simulink model "TST_PT_Grip"  (R2016b)
settings: Solver=FixedStepDiscrete  StartTime=0.0  StopTime=simTime  FixedStep=sampleTime  RelTol=1e-3
values from neighbouring files (symbols this model uses):
  testCase = 1    [initTST_PT_Grip_001.m]    (also in initTST_PT_Grip_002.m = 2)
libraries: simulink x9, UnitTest_Lib x6
settings Model: Creator=zhengjinyan  LastModifiedBy=zhengjinyan
settings DebuggingCC: SignalRangeChecking=error

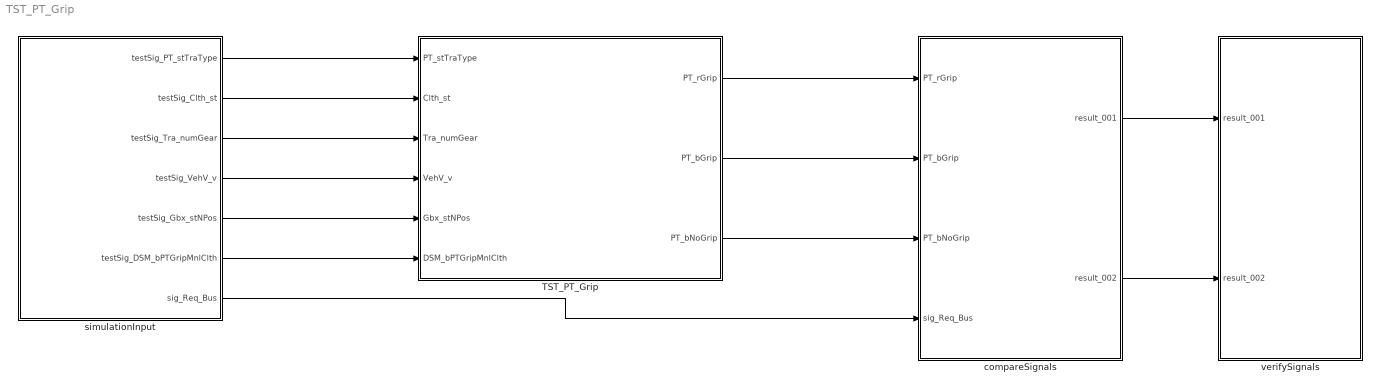
== system TST_PT_Grip ==
  TST_PT_Grip : Subsystem
  compareSignals : Subsystem
  simulationInput : Subsystem
  verifySignals : Subsystem
  wires:
  simulationInput/1(testSig_PT_stTraType) -> TST_PT_Grip/1(PT_stTraType)
  simulationInput/2(testSig_Clth_st) -> TST_PT_Grip/2(Clth_st)
  simulationInput/3(testSig_Tra_numGear) -> TST_PT_Grip/3(Tra_numGear)
  simulationInput/4(testSig_VehV_v) -> TST_PT_Grip/4(VehV_v)
  simulationInput/5(testSig_Gbx_stNPos) -> TST_PT_Grip/5(Gbx_stNPos)
  simulationInput/6(testSig_DSM_bPTGripMnlClth) -> TST_PT_Grip/6(DSM_bPTGripMnlClth)
  TST_PT_Grip/1(PT_rGrip) -> compareSignals/1(PT_rGrip)
  TST_PT_Grip/2(PT_bGrip) -> compareSignals/2(PT_bGrip)
  TST_PT_Grip/3(PT_bNoGrip) -> compareSignals/3(PT_bNoGrip)
  simulationInput/7(sig_Req_Bus) -> compareSignals/4(sig_Req_Bus)
  compareSignals/1(result_001) -> verifySignals/1(result_001)
  compareSignals/2(result_002) -> verifySignals/2(result_002)

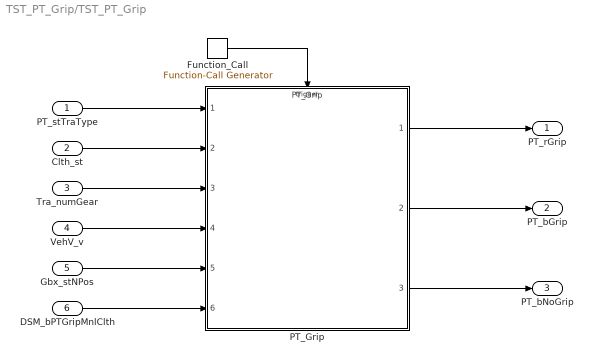
== system TST_PT_Grip/TST_PT_Grip ==
  PT_stTraType : Inport
  Clth_st : Inport  Port=2
  Tra_numGear : Inport  Port=3
  VehV_v : Inport  Port=4
  Gbx_stNPos : Inport  Port=5
  DSM_bPTGripMnlClth : Inport  Port=6
  Function_Call : simulink/Ports & Subsystems/Function-Call Generator  sample_time=sampleTime  numberOfIterations=1
  PT_Grip : ModelReference  ModelNameDialog=PT_Grip  SimulationMode=Normal  ModelReferenceVersion=1.20  TriggerPortName=function  TriggerPortTriggerType=function-call  TriggerPortStatesWhenEnabling=held
  PT_rGrip : Outport
  PT_bGrip : Outport  Port=2
  PT_bNoGrip : Outport  Port=3
  wires:
  Function_Call/1 -> PT_Grip/Trigger
  PT_stTraType/1 -> PT_Grip/1
  Clth_st/1 -> PT_Grip/2
  Tra_numGear/1 -> PT_Grip/3
  VehV_v/1 -> PT_Grip/4
  Gbx_stNPos/1 -> PT_Grip/5
  DSM_bPTGripMnlClth/1 -> PT_Grip/6
  PT_Grip/1 -> PT_rGrip/1
  PT_Grip/2 -> PT_bGrip/1
  PT_Grip/3 -> PT_bNoGrip/1

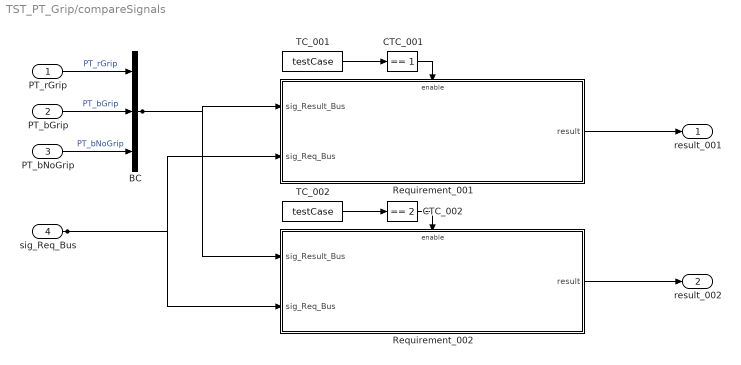
== system TST_PT_Grip/compareSignals ==
  PT_rGrip : Inport
  PT_bGrip : Inport  Port=2
  PT_bNoGrip : Inport  Port=3
  sig_Req_Bus : Inport  Port=4
  BC : BusCreator  Inputs=3
  CTC_001 : simulink/Logic and Bit Operations/Compare To Constant  relop===  const=1  OutDataTypeStr=boolean
  CTC_002 : simulink/Logic and Bit Operations/Compare To Constant  relop===  const=2  OutDataTypeStr=boolean
  Requirement_001 : Subsystem
  Requirement_002 : Subsystem
  TC_001 : Constant  Value=testCase
  TC_002 : Constant  Value=testCase
  result_001 : Outport
  result_002 : Outport  Port=2
  wires:
  PT_rGrip/1 -> BC/1  "PT_rGrip"
  PT_bGrip/1 -> BC/2  "PT_bGrip"
  PT_bNoGrip/1 -> BC/3  "PT_bNoGrip"
  TC_001/1 -> CTC_001/1
  CTC_001/1 -> Requirement_001/Enable
  sig_Req_Bus/1 -> Requirement_001/2(sig_Req_Bus), Requirement_002/2(sig_Req_Bus)
  BC/1 -> Requirement_001/1(sig_Result_Bus), Requirement_002/1(sig_Result_Bus)
  Requirement_001/1(result) -> result_001/1
  TC_002/1 -> CTC_002/1
  CTC_002/1 -> Requirement_002/Enable
  Requirement_002/1(result) -> result_002/1

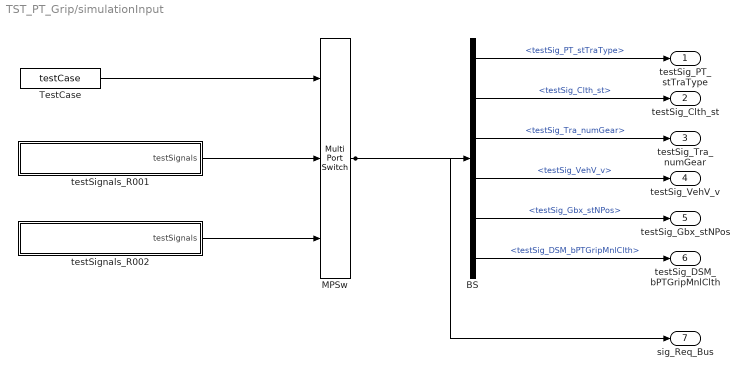
== system TST_PT_Grip/simulationInput ==
  BS : BusSelector  OutputSignals=testSig_PT_stTraType,testSig_Clth_st,testSig_Tra_numGear,testSig_VehV_v,testSig_Gbx_stNPos,testSig_DSM_bPTGripMnlClth
  MPSw : MultiPortSwitch  Inputs=2  SaturateOnIntegerOverflow=on  InputSameDT=on
  TestCase : Constant  Value=testCase
  testSignals_R001 : Subsystem
  testSignals_R002 : Subsystem
  testSig_PT_stTraType : Outport
  testSig_Clth_st : Outport  Port=2
  testSig_Tra_numGear : Outport  Port=3
  testSig_VehV_v : Outport  Port=4
  testSig_Gbx_stNPos : Outport  Port=5
  testSig_DSM_bPTGripMnlClth : Outport  Port=6
  sig_Req_Bus : Outport  Port=7
  wires:
  BS/1 -> testSig_PT_stTraType/1  "<testSig_PT_stTraType>"
  BS/2 -> testSig_Clth_st/1  "<testSig_Clth_st>"
  BS/3 -> testSig_Tra_numGear/1  "<testSig_Tra_numGear>"
  BS/4 -> testSig_VehV_v/1  "<testSig_VehV_v>"
  BS/5 -> testSig_Gbx_stNPos/1  "<testSig_Gbx_stNPos>"
  BS/6 -> testSig_DSM_bPTGripMnlClth/1  "<testSig_DSM_bPTGripMnlClth>"
  MPSw/1 -> BS/1, sig_Req_Bus/1
  TestCase/1 -> MPSw/1
  testSignals_R001/1(testSignals) -> MPSw/2
  testSignals_R002/1(testSignals) -> MPSw/3

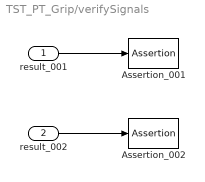
== system TST_PT_Grip/verifySignals ==
  result_001 : Inport
  result_002 : Inport  Port=2
  Assertion_001 : Assertion  Enabled=off
  Assertion_002 : Assertion  Enabled=off
  wires:
  result_001/1 -> Assertion_001/1
  result_002/1 -> Assertion_002/1

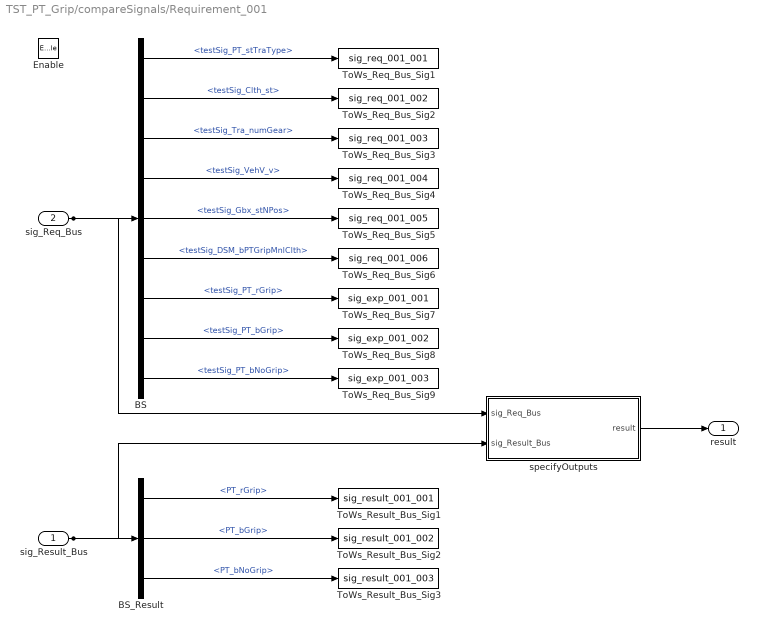
== system TST_PT_Grip/compareSignals/Requirement_001 ==
  sig_Result_Bus : Inport
  sig_Req_Bus : Inport  Port=2
  Enable : EnablePort
  BS : BusSelector  OutputSignals=testSig_PT_stTraType,testSig_Clth_st,testSig_Tra_numGear,testSig_VehV_v,testSig_Gbx_stNPos,testSig_DSM_bPTGripMnlClth,testSig_PT_rGrip,testSig_PT_bGrip,testSig_PT_bNoGrip
  BS_Result : BusSelector  OutputSignals=PT_rGrip,PT_bGrip,PT_bNoGrip
  ToWs_Req_Bus_Sig1 : ToWorkspace  VariableName=sig_req_001_001  SaveFormat=Structure With Time
  ToWs_Req_Bus_Sig2 : ToWorkspace  VariableName=sig_req_001_002  SaveFormat=Structure With Time
  ToWs_Req_Bus_Sig3 : ToWorkspace  VariableName=sig_req_001_003  SaveFormat=Structure With Time
  ToWs_Req_Bus_Sig4 : ToWorkspace  VariableName=sig_req_001_004  SaveFormat=Structure With Time
  ToWs_Req_Bus_Sig5 : ToWorkspace  VariableName=sig_req_001_005  SaveFormat=Structure With Time
  ToWs_Req_Bus_Sig6 : ToWorkspace  VariableName=sig_req_001_006  SaveFormat=Structure With Time
  ToWs_Req_Bus_Sig7 : ToWorkspace  VariableName=sig_exp_001_001  SaveFormat=Structure With Time
  ToWs_Req_Bus_Sig8 : ToWorkspace  VariableName=sig_exp_001_002  SaveFormat=Structure With Time
  ToWs_Req_Bus_Sig9 : ToWorkspace  VariableName=sig_exp_001_003  SaveFormat=Structure With Time
  ToWs_Result_Bus_Sig1 : ToWorkspace  VariableName=sig_result_001_001  SaveFormat=Structure With Time
  ToWs_Result_Bus_Sig2 : ToWorkspace  VariableName=sig_result_001_002  SaveFormat=Structure With Time
  ToWs_Result_Bus_Sig3 : ToWorkspace  VariableName=sig_result_001_003  SaveFormat=Structure With Time
  specifyOutputs : Subsystem
  result : Outport
  wires:
  sig_Req_Bus/1 -> BS/1, specifyOutputs/1(sig_Req_Bus)
  BS/1 -> ToWs_Req_Bus_Sig1/1  "<testSig_PT_stTraType>"
  BS/2 -> ToWs_Req_Bus_Sig2/1  "<testSig_Clth_st>"
  BS/3 -> ToWs_Req_Bus_Sig3/1  "<testSig_Tra_numGear>"
  BS/4 -> ToWs_Req_Bus_Sig4/1  "<testSig_VehV_v>"
  BS/5 -> ToWs_Req_Bus_Sig5/1  "<testSig_Gbx_stNPos>"
  BS/6 -> ToWs_Req_Bus_Sig6/1  "<testSig_DSM_bPTGripMnlClth>"
  BS/7 -> ToWs_Req_Bus_Sig7/1  "<testSig_PT_rGrip>"
  BS/8 -> ToWs_Req_Bus_Sig8/1  "<testSig_PT_bGrip>"
  BS/9 -> ToWs_Req_Bus_Sig9/1  "<testSig_PT_bNoGrip>"
  sig_Result_Bus/1 -> BS_Result/1, specifyOutputs/2(sig_Result_Bus)
  BS_Result/1 -> ToWs_Result_Bus_Sig1/1  "<PT_rGrip>"
  BS_Result/2 -> ToWs_Result_Bus_Sig2/1  "<PT_bGrip>"
  BS_Result/3 -> ToWs_Result_Bus_Sig3/1  "<PT_bNoGrip>"
  specifyOutputs/1(result) -> result/1

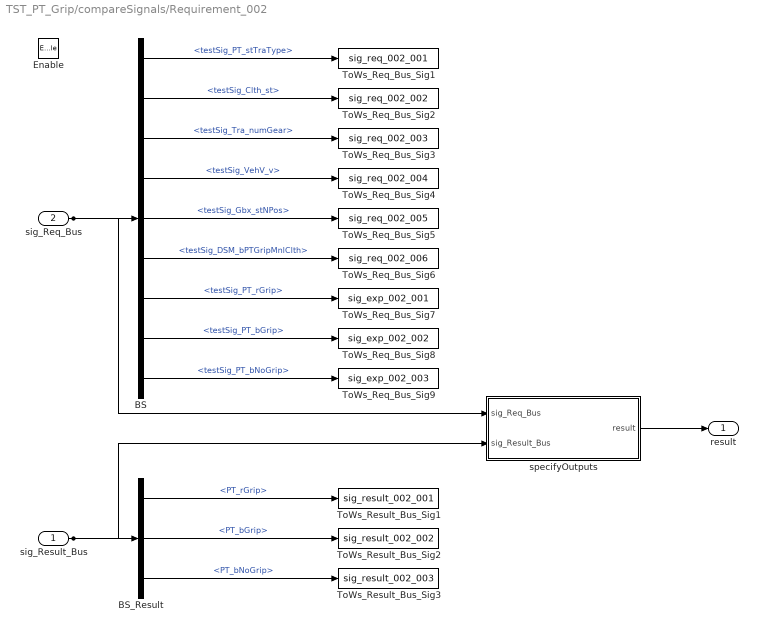
== system TST_PT_Grip/compareSignals/Requirement_002 ==
  sig_Result_Bus : Inport
  sig_Req_Bus : Inport  Port=2
  Enable : EnablePort
  BS : BusSelector  OutputSignals=testSig_PT_stTraType,testSig_Clth_st,testSig_Tra_numGear,testSig_VehV_v,testSig_Gbx_stNPos,testSig_DSM_bPTGripMnlClth,testSig_PT_rGrip,testSig_PT_bGrip,testSig_PT_bNoGrip
  BS_Result : BusSelector  OutputSignals=PT_rGrip,PT_bGrip,PT_bNoGrip
  ToWs_Req_Bus_Sig1 : ToWorkspace  VariableName=sig_req_002_001  SaveFormat=Structure With Time
  ToWs_Req_Bus_Sig2 : ToWorkspace  VariableName=sig_req_002_002  SaveFormat=Structure With Time
  ToWs_Req_Bus_Sig3 : ToWorkspace  VariableName=sig_req_002_003  SaveFormat=Structure With Time
  ToWs_Req_Bus_Sig4 : ToWorkspace  VariableName=sig_req_002_004  SaveFormat=Structure With Time
  ToWs_Req_Bus_Sig5 : ToWorkspace  VariableName=sig_req_002_005  SaveFormat=Structure With Time
  ToWs_Req_Bus_Sig6 : ToWorkspace  VariableName=sig_req_002_006  SaveFormat=Structure With Time
  ToWs_Req_Bus_Sig7 : ToWorkspace  VariableName=sig_exp_002_001  SaveFormat=Structure With Time
  ToWs_Req_Bus_Sig8 : ToWorkspace  VariableName=sig_exp_002_002  SaveFormat=Structure With Time
  ToWs_Req_Bus_Sig9 : ToWorkspace  VariableName=sig_exp_002_003  SaveFormat=Structure With Time
  ToWs_Result_Bus_Sig1 : ToWorkspace  VariableName=sig_result_002_001  SaveFormat=Structure With Time
  ToWs_Result_Bus_Sig2 : ToWorkspace  VariableName=sig_result_002_002  SaveFormat=Structure With Time
  ToWs_Result_Bus_Sig3 : ToWorkspace  VariableName=sig_result_002_003  SaveFormat=Structure With Time
  specifyOutputs : Subsystem
  result : Outport
  wires:
  sig_Req_Bus/1 -> BS/1, specifyOutputs/1(sig_Req_Bus)
  BS/1 -> ToWs_Req_Bus_Sig1/1  "<testSig_PT_stTraType>"
  BS/2 -> ToWs_Req_Bus_Sig2/1  "<testSig_Clth_st>"
  BS/3 -> ToWs_Req_Bus_Sig3/1  "<testSig_Tra_numGear>"
  BS/4 -> ToWs_Req_Bus_Sig4/1  "<testSig_VehV_v>"
  BS/5 -> ToWs_Req_Bus_Sig5/1  "<testSig_Gbx_stNPos>"
  BS/6 -> ToWs_Req_Bus_Sig6/1  "<testSig_DSM_bPTGripMnlClth>"
  BS/7 -> ToWs_Req_Bus_Sig7/1  "<testSig_PT_rGrip>"
  BS/8 -> ToWs_Req_Bus_Sig8/1  "<testSig_PT_bGrip>"
  BS/9 -> ToWs_Req_Bus_Sig9/1  "<testSig_PT_bNoGrip>"
  sig_Result_Bus/1 -> BS_Result/1, specifyOutputs/2(sig_Result_Bus)
  BS_Result/1 -> ToWs_Result_Bus_Sig1/1  "<PT_rGrip>"
  BS_Result/2 -> ToWs_Result_Bus_Sig2/1  "<PT_bGrip>"
  BS_Result/3 -> ToWs_Result_Bus_Sig3/1  "<PT_bNoGrip>"
  specifyOutputs/1(result) -> result/1

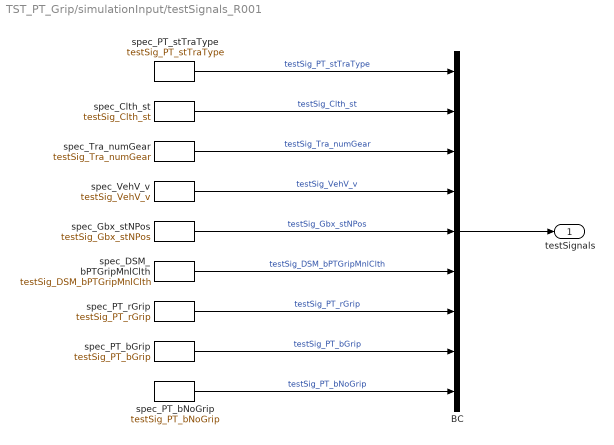
== system TST_PT_Grip/simulationInput/testSignals_R001 ==
  BC : BusCreator  Inputs=9
  spec_Clth_st : FromWorkspace  VariableName=testSig_Clth_st  Interpolate=off  OutputAfterFinalValue=Holding final value
  spec_DSM_bPTGripMnlClth : FromWorkspace  VariableName=testSig_DSM_bPTGripMnlClth  Interpolate=off  OutputAfterFinalValue=Holding final value
  spec_Gbx_stNPos : FromWorkspace  VariableName=testSig_Gbx_stNPos  Interpolate=off  OutputAfterFinalValue=Holding final value
  spec_PT_bGrip : FromWorkspace  VariableName=testSig_PT_bGrip  Interpolate=off  OutputAfterFinalValue=Holding final value
  spec_PT_bNoGrip : FromWorkspace  VariableName=testSig_PT_bNoGrip  Interpolate=off  OutputAfterFinalValue=Holding final value
  spec_PT_rGrip : FromWorkspace  VariableName=testSig_PT_rGrip  Interpolate=off  OutputAfterFinalValue=Holding final value
  spec_PT_stTraType : FromWorkspace  VariableName=testSig_PT_stTraType  Interpolate=off  OutputAfterFinalValue=Holding final value
  spec_Tra_numGear : FromWorkspace  VariableName=testSig_Tra_numGear  Interpolate=off  OutputAfterFinalValue=Holding final value
  spec_VehV_v : FromWorkspace  VariableName=testSig_VehV_v  Interpolate=off  OutputAfterFinalValue=Holding final value
  testSignals : Outport
  wires:
  BC/1 -> testSignals/1
  spec_PT_stTraType/1 -> BC/1  "testSig_PT_stTraType"
  spec_Clth_st/1 -> BC/2  "testSig_Clth_st"
  spec_Tra_numGear/1 -> BC/3  "testSig_Tra_numGear"
  spec_VehV_v/1 -> BC/4  "testSig_VehV_v"
  spec_Gbx_stNPos/1 -> BC/5  "testSig_Gbx_stNPos"
  spec_DSM_bPTGripMnlClth/1 -> BC/6  "testSig_DSM_bPTGripMnlClth"
  spec_PT_rGrip/1 -> BC/7  "testSig_PT_rGrip"
  spec_PT_bGrip/1 -> BC/8  "testSig_PT_bGrip"
  spec_PT_bNoGrip/1 -> BC/9  "testSig_PT_bNoGrip"

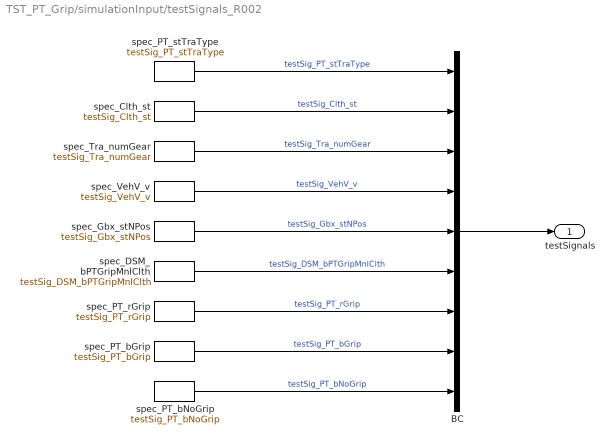
== system TST_PT_Grip/simulationInput/testSignals_R002 ==
  BC : BusCreator  Inputs=9
  spec_Clth_st : FromWorkspace  VariableName=testSig_Clth_st  Interpolate=off  OutputAfterFinalValue=Holding final value
  spec_DSM_bPTGripMnlClth : FromWorkspace  VariableName=testSig_DSM_bPTGripMnlClth  Interpolate=off  OutputAfterFinalValue=Holding final value
  spec_Gbx_stNPos : FromWorkspace  VariableName=testSig_Gbx_stNPos  Interpolate=off  OutputAfterFinalValue=Holding final value
  spec_PT_bGrip : FromWorkspace  VariableName=testSig_PT_bGrip  Interpolate=off  OutputAfterFinalValue=Holding final value
  spec_PT_bNoGrip : FromWorkspace  VariableName=testSig_PT_bNoGrip  Interpolate=off  OutputAfterFinalValue=Holding final value
  spec_PT_rGrip : FromWorkspace  VariableName=testSig_PT_rGrip  Interpolate=off  OutputAfterFinalValue=Holding final value
  spec_PT_stTraType : FromWorkspace  VariableName=testSig_PT_stTraType  Interpolate=off  OutputAfterFinalValue=Holding final value
  spec_Tra_numGear : FromWorkspace  VariableName=testSig_Tra_numGear  Interpolate=off  OutputAfterFinalValue=Holding final value
  spec_VehV_v : FromWorkspace  VariableName=testSig_VehV_v  Interpolate=off  OutputAfterFinalValue=Holding final value
  testSignals : Outport
  wires:
  BC/1 -> testSignals/1
  spec_PT_stTraType/1 -> BC/1  "testSig_PT_stTraType"
  spec_Clth_st/1 -> BC/2  "testSig_Clth_st"
  spec_Tra_numGear/1 -> BC/3  "testSig_Tra_numGear"
  spec_VehV_v/1 -> BC/4  "testSig_VehV_v"
  spec_Gbx_stNPos/1 -> BC/5  "testSig_Gbx_stNPos"
  spec_DSM_bPTGripMnlClth/1 -> BC/6  "testSig_DSM_bPTGripMnlClth"
  spec_PT_rGrip/1 -> BC/7  "testSig_PT_rGrip"
  spec_PT_bGrip/1 -> BC/8  "testSig_PT_bGrip"
  spec_PT_bNoGrip/1 -> BC/9  "testSig_PT_bNoGrip"

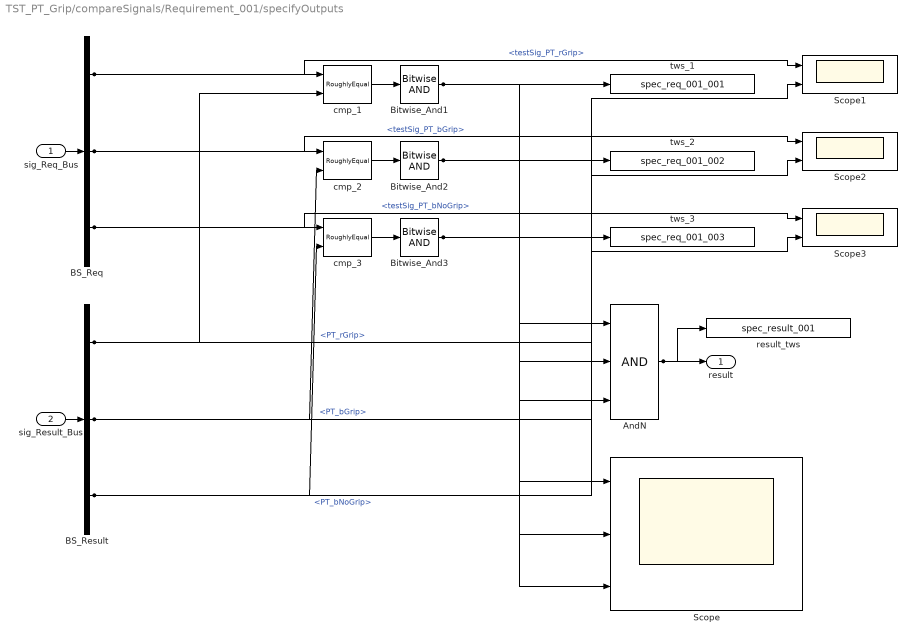
== system TST_PT_Grip/compareSignals/Requirement_001/specifyOutputs ==
  sig_Req_Bus : Inport
  sig_Result_Bus : Inport  Port=2
  AndN : Logic  Inputs=3
  BS_Req : BusSelector  OutputSignals=testSig_PT_rGrip,testSig_PT_bGrip,testSig_PT_bNoGrip
  BS_Result : BusSelector  OutputSignals=PT_rGrip,PT_bGrip,PT_bNoGrip
  Bitwise_And1 : simulink/Logic and Bit Operations/Bitwise Operator  logicop=AND  UseBitMask=off  BitMask=bin2dec('11011001')  BitMaskRealWorld=Stored Integer
  Bitwise_And2 : simulink/Logic and Bit Operations/Bitwise Operator  logicop=AND  UseBitMask=off  BitMask=bin2dec('11011001')  BitMaskRealWorld=Stored Integer
  Bitwise_And3 : simulink/Logic and Bit Operations/Bitwise Operator  logicop=AND  UseBitMask=off  BitMask=bin2dec('11011001')  BitMaskRealWorld=Stored Integer
  Scope : Scope  NumInputPorts=3
  Scope1 : Scope  NumInputPorts=2
  Scope2 : Scope  NumInputPorts=2
  Scope3 : Scope  NumInputPorts=2
  cmp_1 : UnitTest_Lib/RoughlyEqual  slope=0.1
  cmp_2 : UnitTest_Lib/RoughlyEqual  slope=0.1
  cmp_3 : UnitTest_Lib/RoughlyEqual  slope=0.1
  result_tws : ToWorkspace  VariableName=spec_result_001
  tws_1 : ToWorkspace  VariableName=spec_req_001_001
  tws_2 : ToWorkspace  VariableName=spec_req_001_002
  tws_3 : ToWorkspace  VariableName=spec_req_001_003
  result : Outport
  wires:
  sig_Req_Bus/1 -> BS_Req/1
  sig_Result_Bus/1 -> BS_Result/1
  AndN/1 -> result/1, result_tws/1
  BS_Req/1 -> cmp_1/1, Scope1/1  "<testSig_PT_rGrip>"
  BS_Result/1 -> cmp_1/2, Scope1/2  "<PT_rGrip>"
  cmp_1/1 -> Bitwise_And1/1
  Bitwise_And1/1 -> tws_1/1, AndN/1, Scope/1
  BS_Req/2 -> cmp_2/1, Scope2/1  "<testSig_PT_bGrip>"
  BS_Result/2 -> cmp_2/2, Scope2/2  "<PT_bGrip>"
  cmp_2/1 -> Bitwise_And2/1
  Bitwise_And2/1 -> tws_2/1, AndN/2, Scope/2
  BS_Req/3 -> cmp_3/1, Scope3/1  "<testSig_PT_bNoGrip>"
  BS_Result/3 -> cmp_3/2, Scope3/2  "<PT_bNoGrip>"
  cmp_3/1 -> Bitwise_And3/1
  Bitwise_And3/1 -> tws_3/1, AndN/3, Scope/3

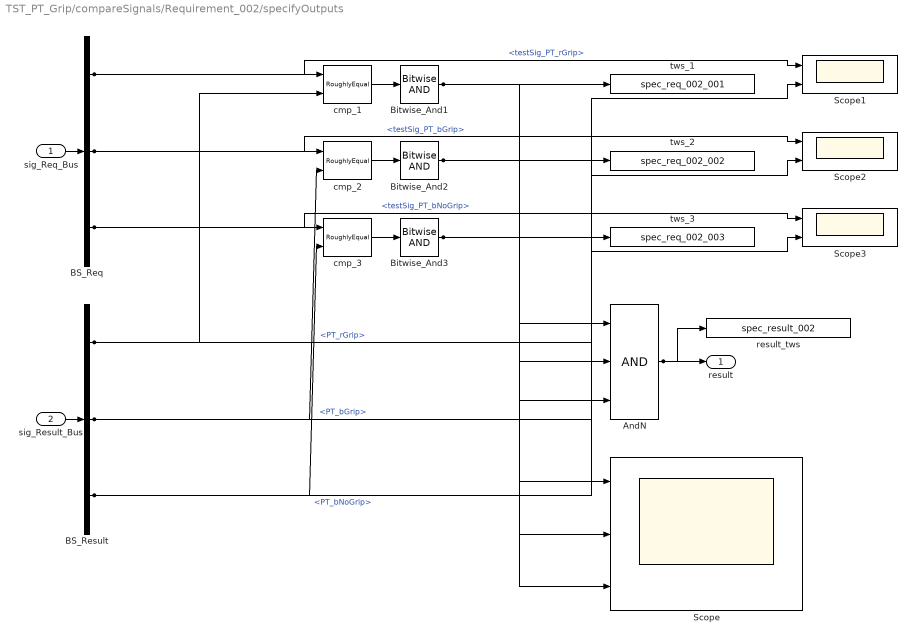
== system TST_PT_Grip/compareSignals/Requirement_002/specifyOutputs ==
  sig_Req_Bus : Inport
  sig_Result_Bus : Inport  Port=2
  AndN : Logic  Inputs=3
  BS_Req : BusSelector  OutputSignals=testSig_PT_rGrip,testSig_PT_bGrip,testSig_PT_bNoGrip
  BS_Result : BusSelector  OutputSignals=PT_rGrip,PT_bGrip,PT_bNoGrip
  Bitwise_And1 : simulink/Logic and Bit Operations/Bitwise Operator  logicop=AND  UseBitMask=off  BitMask=bin2dec('11011001')  BitMaskRealWorld=Stored Integer
  Bitwise_And2 : simulink/Logic and Bit Operations/Bitwise Operator  logicop=AND  UseBitMask=off  BitMask=bin2dec('11011001')  BitMaskRealWorld=Stored Integer
  Bitwise_And3 : simulink/Logic and Bit Operations/Bitwise Operator  logicop=AND  UseBitMask=off  BitMask=bin2dec('11011001')  BitMaskRealWorld=Stored Integer
  Scope : Scope  NumInputPorts=3
  Scope1 : Scope  NumInputPorts=2
  Scope2 : Scope  NumInputPorts=2
  Scope3 : Scope  NumInputPorts=2
  cmp_1 : UnitTest_Lib/RoughlyEqual  slope=0.1
  cmp_2 : UnitTest_Lib/RoughlyEqual  slope=0.1
  cmp_3 : UnitTest_Lib/RoughlyEqual  slope=0.1
  result_tws : ToWorkspace  VariableName=spec_result_002
  tws_1 : ToWorkspace  VariableName=spec_req_002_001
  tws_2 : ToWorkspace  VariableName=spec_req_002_002
  tws_3 : ToWorkspace  VariableName=spec_req_002_003
  result : Outport
  wires:
  sig_Req_Bus/1 -> BS_Req/1
  sig_Result_Bus/1 -> BS_Result/1
  AndN/1 -> result/1, result_tws/1
  BS_Req/1 -> cmp_1/1, Scope1/1  "<testSig_PT_rGrip>"
  BS_Result/1 -> cmp_1/2, Scope1/2  "<PT_rGrip>"
  cmp_1/1 -> Bitwise_And1/1
  Bitwise_And1/1 -> tws_1/1, AndN/1, Scope/1
  BS_Req/2 -> cmp_2/1, Scope2/1  "<testSig_PT_bGrip>"
  BS_Result/2 -> cmp_2/2, Scope2/2  "<PT_bGrip>"
  cmp_2/1 -> Bitwise_And2/1
  Bitwise_And2/1 -> tws_2/1, AndN/2, Scope/2
  BS_Req/3 -> cmp_3/1, Scope3/1  "<testSig_PT_bNoGrip>"
  BS_Result/3 -> cmp_3/2, Scope3/2  "<PT_bNoGrip>"
  cmp_3/1 -> Bitwise_And3/1
  Bitwise_And3/1 -> tws_3/1, AndN/3, Scope/3
